simulink model "TCMSSystem"  (R2019b)
settings: configuration reference "ConfigSet_TCMSSystem_Reference" (kept outside this file)
model workspace (MAT data in the model file):
  Prm_TCMSSystem : Simulink.Parameter (value not decoded)
  SampleTime = 0.05
symbols that are objects in the model workspace (value not decoded): Prm_TCMSSystem
undefined symbols (not defined in the file): ADDIntervention, AK1Status, AK2Status, AKContactorStatus, AllDoorsClosed, AllLeftDoorsClosed, AllRightDoorsClosed, APS1Fault, APS1Isolated, APS1OutputVoltage, APS1Status, APS2Fault, APS2Isolated, APS2OutputVoltage, APS2Status, APSKAKContactor, ASCOEnd1, ASCOEnd2, ATBMode, ATCBypassMode, ATCStatusNotOK, ATOMode, ATPLowSpeedCutoutStatus, ATPMode, AuxCompressor, BatteryCurrent, BatteryIsolationContactor, BatteryTemperature, BatteryVoltage, BCG1Fault, BCG1Isolated, BCG1IsolationFailed, BCG1OutputCurrent, BCG1Status, BCG2Fault, BCG2Isolated, BCG2OutputCurrent, BCG2Status, BCGOutputVoltage, BECU1AxleLockedWheelSet1, BECU2AxleLockedWheelSet2, BECUFaulty, BECUMajorFault, BECUMinorFault, BECUStatus, BIC1Inside, BIC1Outside, BIC2Inside, BIC2Outside, Bogie, Bogie1WSPStatus, Bogie2WSPStatus, BogieFaulty, BogieIsolationStatus, BogieSupportedMass, BrakeCylinderPressureGauge, BrakeLoopCBTripped, BrakeLoopOpenTL, BrakeTrainLineStatus, BrakingDemand ... (+215)
libraries: TimersLib x257, simulink x137, LatchesLib x42, VectorOperationsLib x15, TestBenchLib x12, MathOperationsLib x2, FiltersLib x1
(part 2 of 16)

== system TCMSSystem/TCMSSystemPerVehicle/EnabledTCMSVehicle/OutputsPacking/TCMSControlOutputs ==
  PangraphOut : Inport
  TractionOut : Inport  Port=2
  DoorsOut : Inport  Port=3
  ElectricalOut : Inport  Port=4
  PneumaticOut : Inport  Port=5
  Bus Assignment2 : BusAssignment  AssignedSignals=PantographSystem,TractionSBraking,DoorSystem,ElectricalSystem,PneumaticSystem
  Constant1 : Constant  Value=0  OutDataTypeStr=Bus: BD_TCMSSystem_Out_Vehicle_Control
  TCMSControlOut : Outport
  wires:
  Bus Assignment2/1 -> TCMSControlOut/1  "TCMSControlOut"
  Constant1/1 -> Bus Assignment2/1
  TractionOut/1 -> Bus Assignment2/3
  DoorsOut/1 -> Bus Assignment2/4
  PangraphOut/1 -> Bus Assignment2/2
  ElectricalOut/1 -> Bus Assignment2/5
  PneumaticOut/1 -> Bus Assignment2/6

== system TCMSSystem/TCMSSystemPerVehicle/EnabledTCMSVehicle/OutputsPacking/TCMSDisplayOutputs ==
  PangraphOut : Inport
  TractionBrakingOut : Inport  Port=2
  PneumaticsOut : Inport  Port=3
  DoorsOut : Inport  Port=4
  ElectricalOut : Inport  Port=5
  TCMSFaults : Inport  Port=6
  TCMSSystem : Inport  Port=7
  VehicleLevelFaults : Inport  Port=8
  ElectricalControls : Inport  Port=9
  DoorsControl : Inport  Port=10
  TractionControl : Inport  Port=11
  PneumaticsControl : Inport  Port=12
  Enable : EnablePort
  Bus Assignment1 : BusAssignment  AssignedSignals=PantographSystem,TractionBraking,PneumaticsSystem,DoorSystem,ElectricalSystem,TCMSSystem
  Constant2 : Constant  Value=0  OutDataTypeStr=Bus: BD_TCMSSystem_Out_Vehicle_Display
  TCMSMessageEvents : Subsystem
  TCMSControlDisplay : Outport
  wires:
  DoorsOut/1 -> Bus Assignment1/5
  Constant2/1 -> Bus Assignment1/1
  PangraphOut/1 -> Bus Assignment1/2
  TractionBrakingOut/1 -> Bus Assignment1/3
  PneumaticsOut/1 -> Bus Assignment1/4
  Bus Assignment1/1 -> TCMSMessageEvents/1(BusIn)  "TCMSControlDisplay"
  ElectricalOut/1 -> Bus Assignment1/6
  TCMSMessageEvents/1(BusOut) -> TCMSControlDisplay/1
  TCMSFaults/1 -> TCMSMessageEvents/2(TCMSFaults)
  TCMSSystem/1 -> Bus Assignment1/7
  VehicleLevelFaults/1 -> TCMSMessageEvents/4(VehicleLevelFaults)
  ElectricalControls/1 -> TCMSMessageEvents/5(ElectricalControl)
  DoorsControl/1 -> TCMSMessageEvents/6(DoorsControl)
  TractionControl/1 -> TCMSMessageEvents/7(TractionControl)
  PneumaticsControl/1 -> TCMSMessageEvents/3(PneumaticsControl)

== system TCMSSystem/TCMSSystemPerVehicle/EnabledTCMSVehicle/TCMSDoors/CabControlsExtract ==
  TCMSConfig : Inport
  ElectricalSignals : Inport  Port=2
  CBTCSignals : Inport  Port=3
  AND : Logic  AllPortsSameDT=off  OutDataTypeStr=boolean
  Bus Selector : BusSelector  OutputSignals=CabActive
  Bus Selector1 : BusSelector  OutputSignals=HasCab
  CabActiveTrainControl : Subsystem  TreatAsAtomicUnit=on
  CabInactiveNoTrainControl : Subsystem  TreatAsAtomicUnit=on
  Data Type Conversion : DataTypeConversion  OutDataTypeStr=uint32
  If : If
  Merge : Merge
  DoorsTrainWireSource : Outport
  wires:
  Bus Selector/1 -> AND/2  "<CabActive>"
  AND/1 -> Data Type Conversion/1
  If/2 -> CabInactiveNoTrainControl/Action
  Bus Selector1/1 -> AND/1  "<HasCab>"
  ElectricalSignals/1 -> Bus Selector/1
  TCMSConfig/1 -> Bus Selector1/1
  If/1 -> CabActiveTrainControl/Action
  Merge/1 -> DoorsTrainWireSource/1  "DoorsTrainWireSource"
  Data Type Conversion/1 -> If/1
  CabInactiveNoTrainControl/1(Out1) -> Merge/2
  CabActiveTrainControl/1(Out1) -> Merge/1
  CBTCSignals/1 -> CabActiveTrainControl/1(CBTC)

== system TCMSSystem/TCMSSystemPerVehicle/EnabledTCMSVehicle/TCMSDoors/DoorsControl ==
  In Bus Element4 : Inport  PortName=DisplayControl  Element=RightDoorsEmergencyReleaseCommand
  In Bus Element5 : Inport  PortName=DisplayControl  Element=LeftDoorsEmergencyReleaseCommand
  In Bus Element6 : Inport  PortName=DisplayControl  Element=DoorA1IsolateVDUReq
  In Bus Element16 : Inport  PortName=DisplayControl  Element=DoorA2IsolateVDUReq
  In Bus Element17 : Inport  PortName=DisplayControl  Element=DoorA3IsolateVDUReq
  In Bus Element18 : Inport  PortName=DisplayControl  Element=DoorA4IsolateVDUReq
  In Bus Element19 : Inport  PortName=DisplayControl  Element=DoorB1IsolateVDUReq
  In Bus Element21 : Inport  PortName=DisplayControl  Element=DoorB2IsolateVDUReq
  In Bus Element26 : Inport  PortName=DisplayControl  Element=DoorB3IsolateVDUReq
  In Bus Element27 : Inport  PortName=DisplayControl  Element=DoorB4IsolateVDUReq
  In Bus Element14 : Inport  Port=2  PortName=ElectricalSignals  Element=LeftDoorOpen
  In Bus Element15 : Inport  Port=2  PortName=ElectricalSignals  Element=RightDoorOpen
  In Bus Element22 : Inport  Port=2  PortName=ElectricalSignals  Element=LeftDoorClose
  In Bus Element23 : Inport  Port=2  PortName=ElectricalSignals  Element=RightDoorClose
  In Bus Element24 : Inport  Port=2  PortName=ElectricalSignals  Element=LeftDoorRelease
  In Bus Element25 : Inport  Port=2  PortName=ElectricalSignals  Element=RightDoorRelease
  In Bus Element7 : Inport  Port=3  PortName=DoorWireStates  Element=LeftDoorOpenRequest
  In Bus Element8 : Inport  Port=3  PortName=DoorWireStates  Element=RightDoorOpenRequest
  In Bus Element9 : Inport  Port=3  PortName=DoorWireStates  Element=LeftDoorCloseRequest
  In Bus Element20 : Inport  Port=3  PortName=DoorWireStates  Element=RightDoorCloseRequest
  In4 : Inport  Port=4
  Bus Assignment : BusAssignment  AssignedSignals=RightDoorEmergencyRelease,LeftDoorEmergencyRelease,DoorLeft1Isolation,DoorLeft2Isolation,DoorLeft3Isolation,DoorLeft4Isolation,DoorRight1Isolation,DoorRight2Isolation,DoorRight3Isolation,DoorRight4Isolation,LeftSideDoorOpenRequest,RightSideDoorOpenRequest,LeftSideDoorCloseRequest,RightSideDoorCloseRequest,LeftSideDoorRelease,RightSideDoorRelease
  Bus Selector : BusSelector  OutputSignals=Orientation
  Constant7 : Constant  Value=0  OutDataTypeStr=Bus: BD_TCMSSystem_Out_Vehicle_Control_DoorSystem
  Data Type Conversion{1..10} (10 alike) : DataTypeConversion  OutDataTypeStr=boolean
  Demux10 : Demux
  Demux9 : Demux
  For Each Subsystem4 : Subsystem  TreatAsAtomicUnit=on
  OR{,1..3} (4 alike) : Logic  Operator=OR  AllPortsSameDT=off  OutDataTypeStr=boolean
  TimerOffDelay NoInit{,1..3} (4 alike) : TimersLib/TimerOffDelay NoInit  UpperSaturationLimit=0.5  SampleTime=-1
      settings: SourceProductName=Sydac Utilities
  Vector Concatenate4 : Concatenate  NumInputs=4
  Vector Concatenate5 : Concatenate  NumInputs=4
  Control : Outport
  wires:
  Bus Assignment/1 -> Control/1  "Control"
  Constant7/1 -> Bus Assignment/1  "Control"
  In Bus Element4/1 -> Data Type Conversion4/1
  In Bus Element5/1 -> Data Type Conversion1/1
  Data Type Conversion4/1 -> Bus Assignment/2
  Data Type Conversion1/1 -> Bus Assignment/3
  In Bus Element14/1 -> OR/1
  In Bus Element7/1 -> TimerOffDelay NoInit/1
  In Bus Element22/1 -> OR1/1
  In Bus Element9/1 -> TimerOffDelay NoInit2/1
  In Bus Element15/1 -> OR2/1
  In Bus Element8/1 -> TimerOffDelay NoInit1/1
  In Bus Element20/1 -> TimerOffDelay NoInit3/1
  In Bus Element23/1 -> OR3/1
  Demux9/1 -> Data Type Conversion2/1
  Demux9/2 -> Data Type Conversion3/1
  Demux9/3 -> Data Type Conversion5/1
  Demux9/4 -> Data Type Conversion7/1
  Demux10/1 -> Data Type Conversion8/1
  Demux10/2 -> Data Type Conversion9/1
  Demux10/3 -> Data Type Conversion10/1
  Demux10/4 -> Data Type Conversion6/1
  OR/1 -> Bus Assignment/12
  OR2/1 -> Bus Assignment/13
  OR1/1 -> Bus Assignment/14
  OR3/1 -> Bus Assignment/15
  In Bus Element24/1 -> Bus Assignment/16
  In Bus Element25/1 -> Bus Assignment/17
  TimerOffDelay NoInit/1 -> OR/2
  TimerOffDelay NoInit1/1 -> OR2/2
  TimerOffDelay NoInit2/1 -> OR1/2
  TimerOffDelay NoInit3/1 -> OR3/2
  For Each Subsystem4/1(WireState1) -> Demux9/1
  For Each Subsystem4/2(WireState2) -> Demux10/1
  Vector Concatenate5/1 -> For Each Subsystem4/2(Source2)
  Bus Selector/1 -> For Each Subsystem4/3(Orientation)  "<Orientation>"
  Vector Concatenate4/1 -> For Each Subsystem4/1(Source1)
  In Bus Element6/1 -> Vector Concatenate4/1
  In Bus Element16/1 -> Vector Concatenate4/2
  In Bus Element17/1 -> Vector Concatenate4/3
  In Bus Element18/1 -> Vector Concatenate4/4
  In Bus Element19/1 -> Vector Concatenate5/1
  In Bus Element21/1 -> Vector Concatenate5/2
  In Bus Element26/1 -> Vector Concatenate5/3
  In Bus Element27/1 -> Vector Concatenate5/4
  In4/1 -> Bus Selector/1
  Data Type Conversion2/1 -> Bus Assignment/4
  Data Type Conversion3/1 -> Bus Assignment/5
  Data Type Conversion5/1 -> Bus Assignment/6
  Data Type Conversion7/1 -> Bus Assignment/7
  Data Type Conversion6/1 -> Bus Assignment/11
  Data Type Conversion8/1 -> Bus Assignment/8
  Data Type Conversion9/1 -> Bus Assignment/9
  Data Type Conversion10/1 -> Bus Assignment/10

== system TCMSSystem/TCMSSystemPerVehicle/EnabledTCMSVehicle/TCMSDoors/DoorsDisplay ==
  CommonVehicleConfig : Inport
  TCMSSystemVehicleConfig : Inport  Port=2
  In Bus Element12 : Inport  Port=3  PortName=ElectricalSignals
  In Bus Element13 : Inport  Port=3  PortName=ElectricalSignals  Element=EmergencyDoorNotOpenStatus
  DoorSystem : Inport  Port=4
  In Bus Element11 : Inport  Port=5  PortName=InputControlStates
  In Bus Element1 : Inport  Port=5  PortName=InputControlStates  Element=CabSaloonPartitionDoorOpen
  In Bus Element2 : Inport  Port=5  PortName=InputControlStates  Element=EmergencyDoorCoverRemoved
  In Bus Element : Inport  Port=5  PortName=InputControlStates  Element=DoorLoopBypassActive
  In Bus Element3 : Inport  Port=5  PortName=InputControlStates  Element=LeftDoor1Lockout
  In Bus Element4 : Inport  Port=5  PortName=InputControlStates  Element=LeftDoor2Lockout
  In Bus Element5 : Inport  Port=5  PortName=InputControlStates  Element=LeftDoor3Lockout
  In Bus Element6 : Inport  Port=5  PortName=InputControlStates  Element=LeftDoor4Lockout
  In Bus Element7 : Inport  Port=5  PortName=InputControlStates  Element=RightDoor1Lockout
  In Bus Element8 : Inport  Port=5  PortName=InputControlStates  Element=RightDoor2Lockout
  In Bus Element9 : Inport  Port=5  PortName=InputControlStates  Element=RightDoor3Lockout
  In Bus Element10 : Inport  Port=5  PortName=InputControlStates  Element=RightDoor4Lockout
  AND : Logic  AllPortsSameDT=off  OutDataTypeStr=boolean
  AND2 : Logic  Operator=NOT  AllPortsSameDT=off  OutDataTypeStr=boolean
  AND3 : Logic  AllPortsSameDT=off  OutDataTypeStr=boolean
  Bus Assignment : BusAssignment  AssignedSignals=AllRightDoorsClosed,AllLeftDoorsClosed,AllDoorsClosed,Doors,EmerDoorFaultMessage,EmergencyEscapeDoorLocked,UnexpectedDoorOpeningDetectedByCC,EmergencyEscapeDoorOpen
  Bus Assignment1 : BusAssignment  AssignedSignals=CabSaloonPartitionDoorOpen,EmergencyDoorCoverRemoved,DoorLoopBypassActive,LeftDoor1Lockout,LeftDoor2Lockout,LeftDoor3Lockout,LeftDoor4Lockout,RightDoor1Lockout,RightDoor2Lockout,RightDoor3Lockout,RightDoor4Lockout
  Bus Selector : BusSelector  OutputSignals=AllRightDoorsClosed,AllLeftDoorsClosed,AllDoorsClosed
  Bus Selector1 : BusSelector  OutputSignals=EmergencyDoor.EmerDoorOpenFaultMessage,EmergencyDoor.EmergencyDoorLocked
  Bus Selector2 : BusSelector  OutputSignals=HasCab
  CabTrainDisplay : Subsystem
  Constant7 : Constant  Value=0  OutDataTypeStr=Bus: BD_TCMSSystem_Out_Vehicle_Display_DoorSystem
  Data Type Conversion{,2..4} (4 alike) : DataTypeConversion
  TCMSVehicleInfo : Subsystem
  Display : Outport
  wires:
  TCMSVehicleInfo/1(TCMSVehicleInfo) -> Bus Assignment/5  "TCMSVehicleInfo"
  DoorSystem/1 -> Bus Selector1/1, TCMSVehicleInfo/1(DoorSystem)
  Bus Selector/1 -> Bus Assignment/2  "<AllRightDoorsClosed>"
  Bus Selector/2 -> Bus Assignment/3  "<AllLeftDoorsClosed>"
  Bus Selector/3 -> Bus Assignment/4  "<AllDoorsClosed>"
  CabTrainDisplay/1(CabTrainDisplay) -> Bus Selector/1  "CabTrainDisplay"
  In Bus Element12/1 -> TCMSVehicleInfo/3(ElectricalSignals), CabTrainDisplay/2(ElectricalSignals)
  TCMSSystemVehicleConfig/1 -> Bus Selector2/1, CabTrainDisplay/1(TCMSConfig)
  Bus Assignment1/1 -> Display/1  "Display"
  Constant7/1 -> Bus Assignment/1  "Display"
  Bus Selector1/2 -> AND3/2  "<EmergencyDoorLocked>"
  Data Type Conversion/1 -> Bus Assignment/6
  CommonVehicleConfig/1 -> TCMSVehicleInfo/2(CommonVehicleConfig)
  Bus Selector1/1 -> AND/2  "<EmerDoorOpenFaultMessage>"
  Bus Selector2/1 -> [HasCab]  "<HasCab>"
  AND/1 -> Data Type Conversion/1
  [HasCab] -> AND/1, AND3/1
  Data Type Conversion3/1 -> Bus Assignment/7
  AND3/1 -> Data Type Conversion3/1
  TCMSVehicleInfo/2(UnexpectedDoorOpened) -> Data Type Conversion4/1
  Data Type Conversion4/1 -> Bus Assignment/8
  In Bus Element11/1 -> TCMSVehicleInfo/4(InputControlStates)
  Bus Assignment/1 -> Bus Assignment1/1  "Display"
  In Bus Element9/1 -> Bus Assignment1/11
  In Bus Element5/1 -> Bus Assignment1/7
  In Bus Element7/1 -> Bus Assignment1/9
  In Bus Element6/1 -> Bus Assignment1/8
  In Bus Element2/1 -> Bus Assignment1/3
  In Bus Element4/1 -> Bus Assignment1/6
  In Bus Element/1 -> Bus Assignment1/4
  In Bus Element1/1 -> Bus Assignment1/2
  In Bus Element8/1 -> Bus Assignment1/10
  In Bus Element3/1 -> Bus Assignment1/5
  In Bus Element10/1 -> Bus Assignment1/12
  In Bus Element13/1 -> AND2/1
  Data Type Conversion2/1 -> Bus Assignment/9
  AND2/1 -> Data Type Conversion2/1
